simulink model "DCMotorClosedLoopControl"  (R2021a)
settings: Solver=VariableStepAuto  StartTime=0.0  StopTime=10.0  RelTol=1e-3
settings Model: Creator=Sanjeev  LastModifiedBy=Sanjeev

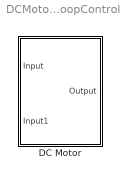
== system DCMotorClosedLoopControl ==
  DC Motor : Subsystem

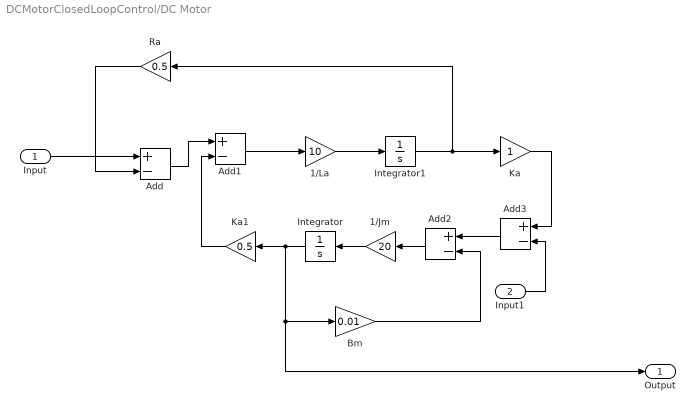
== system DCMotorClosedLoopControl/DC Motor ==
  Input : Inport
  Input1 : Inport  Port=2
  1/Jm : Gain  Gain=20
  1/La : Gain  Gain=10
  Add{,1..3} (4 alike) : Sum  Inputs=+-
  Bm : Gain  Gain=0.01
  Integrator : Integrator
  Integrator1 : Integrator
  Ka : Gain
  Ka1 : Gain  Gain=0.5
  Ra : Gain  Gain=0.5
  Output : Outport
  wires:
  Ka/1 -> Add3/1
  1/Jm/1 -> Integrator/1
  Input/1 -> Add/1
  Ka1/1 -> Add1/2
  Ra/1 -> Add/2
  Add2/1 -> 1/Jm/1
  Integrator1/1 -> Ka/1, Ra/1
  Integrator/1 -> Ka1/1, Output/1, Bm/1
  Bm/1 -> Add2/2
  Input1/1 -> Add3/2
  Add/1 -> Add1/1
  Add1/1 -> 1/La/1
  Add3/1 -> Add2/1
  1/La/1 -> Integrator1/1
